simulink model "parte4_1"  (R2021b)
settings: Solver=FixedStepDiscrete  StartTime=0.0  StopTime=20  FixedStep=.03  RelTol=1e-3  EnableMultiTasking=on
PostLoadFcn:
  | try,
  | codertarget.arduinobase.registry.setBaudRate(gcs,115200)
  | disp('baud rate set to 115200 for external mode hardware serial')
  | baudrate='set_to_115200'
  | catch
  | disp('baud rate setting not needed in this version')
  | end
undefined symbols (not defined in the file): DiscIntNeverNeededParam, EncCov, h, L, Lc
libraries: MinSegLibrary_M2V5 x2, simulink x1
settings Model: SimulationMode=external  ExtModeTrigDuration=2  Creator=Alec  LastModifiedBy=Dylan
settings SolverCC: AlgebraicLoopSolver=TrustRegion
settings DataIOCC: LimitDataPoints=on  SaveFormat=Array  ReturnWorkspaceOutputs=off
settings OptimizationCC: EnhancedBackFolding=on  PassReuseOutputArgsAs=Individual arguments  ExpressionDepthLimit=2147483647  ZeroExternalMemoryAtStartup=off  ZeroInternalMemoryAtStartup=off  MaxStackSize=64  OptimizeBlockOrder=speed  DifferentSizesBufferReuse=on  OptimizationCustomize=off  EfficientTunableParamExpr=on
settings DebuggingCC: UnderspecifiedInitializationDetection=Classic  MergeDetectMultiDrivingBlocksExec=none  ParameterTunabilityLossMsg=error  StateNameClashWarn=warning  SFUnexpectedBacktrackingDiag=warning  SFNoUnconditionalDefaultTransitionDiag=warning  SFExecutionAtInitializationDiag=none  SFMachineParentedDataDiag=warning  ArithmeticOperatorsInVariantConditions=warning
settings HardwareCC: ProdBitPerInt=16  ProdBitPerPointer=16  ProdBitPerSizeT=16  ProdBitPerPtrDiffT=16  ProdLargestAtomicFloat=None  ProdWordSize=8  ProdHWDeviceType=Atmel->AVR
settings ModelReferenceCC: PropagateSignalLabelsOutOfModel=off
settings SFSimCC: SimUseLocalCustomCode=off  MATLABDynamicMemAlloc=off  CustomCodeUndefinedFunction=UseInterfaceOnly
settings RTWCC: Description=Embedded Coder  SystemTargetFile=ert.tlc  HardwareBoard=Arduino Mega 2560  TemplateMakefile=ert_default_tmf  RTWVerbose=off  RTWUseLocalCustomCode=off  Toolchain=Arduino AVR  BuildConfiguration=Faster Runs
settings CodeAppCC: ForceParamTrailComments=on  IgnoreCustomStorageClasses=off  OperatorAnnotations=on  SimulinkDataObjDesc=on  SFDataObjDesc=on  CustomSymbolStrType=$N$R$M  InsertBlockDesc=on  InternalIdentifier=Classic
settings ERTTargetCC: SupportContinuousTime=on  SupportVariableSizeSignals=on  ExtModeTransport=3  ExtModeStaticAlloc=on  ExtModeStaticAllocSize=2048  ExtModeMexFile=ext_xcp  ExtModeIntrfLevel=Level2 - Open
settings ConfigComp: CovMetricSettings=dw  CovSaveCumulativeToWorkspaceVar=on  CovSaveSingleToWorkspaceVar=on  CovExternalEMLEnable=off

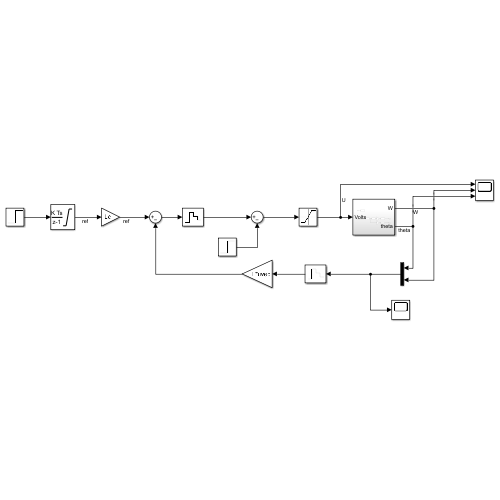
[thumbnail: Simulink's stored preview of the top-level diagram]
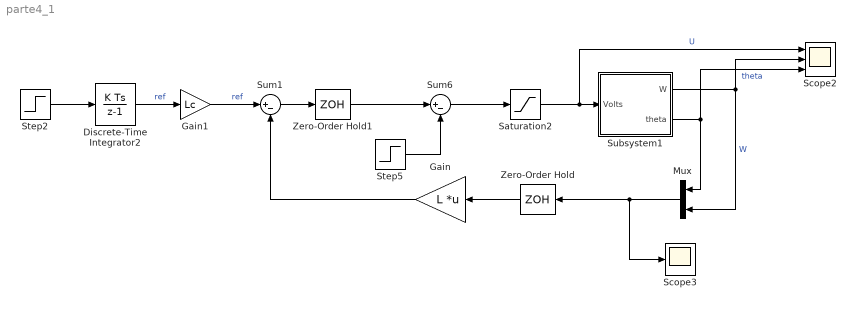
== system parte4_1 ==
  Discrete-Time Integrator2 : DiscreteIntegrator  SampleTime=h  LimitOutput=on  UpperSaturationLimit=50  LowerSaturationLimit=-50  ICPrevOutput=DiscIntNeverNeededParam  ICPrevScaledInput=DiscIntNeverNeededParam
  Gain : Gain  Gain=L  Multiplication=Matrix(K*u) (u vector)
  Gain1 : Gain  Gain=Lc
  Mux : Mux  Inputs=2
  Saturation2 : Saturate  UpperLimit=4.8  LowerLimit=-4.8
  Scope2 : Scope  NumInputPorts=3
  Scope3 : Scope
  Step2 : Step  After=60  SampleTime=0
  Step5 : Step  Time=10  After=2  SampleTime=0
  Subsystem1 : Subsystem
  Sum1 : Sum  Inputs=|+-
  Sum6 : Sum  Inputs=|+-
  Zero-Order Hold : ZeroOrderHold  SampleTime=h
  Zero-Order Hold1 : ZeroOrderHold  SampleTime=h
  wires:
  Subsystem1/2(theta) -> Mux/1, Scope2/3  "theta"
  Gain/1 -> Sum1/2
  Zero-Order Hold/1 -> Gain/1
  Step2/1 -> Discrete-Time Integrator2/1
  Saturation2/1 -> Subsystem1/1(Volts), Scope2/1  "U"
  Discrete-Time Integrator2/1 -> Gain1/1  "ref"
  Zero-Order Hold1/1 -> Sum6/1
  Subsystem1/1(W) -> Mux/2, Scope2/2  "W"
  Step5/1 -> Sum6/2
  Mux/1 -> Scope3/1, Zero-Order Hold/1
  Gain1/1 -> Sum1/1  "ref"
  Sum6/1 -> Saturation2/1
  Sum1/1 -> Zero-Order Hold1/1

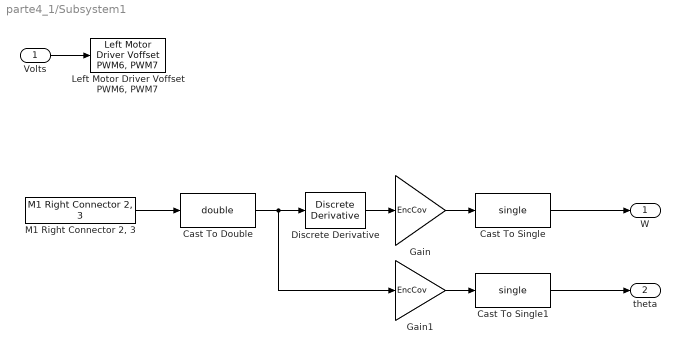
== system parte4_1/Subsystem1 ==
  Volts : Inport
  Cast To Double : DataTypeConversion  OutDataTypeStr=double
  Cast To Single : DataTypeConversion  OutDataTypeStr=single
  Cast To Single1 : DataTypeConversion  OutDataTypeStr=single
  Discrete Derivative : simulink/Discrete/Discrete Derivative  gainval=1.0  ICPrevScaledInput=0.0  OutMin=[]  OutMax=[]  OutDataType=fixdt(1, 16)  OutScaling=2^-10  DoSatur=off
  Gain : Gain  Gain=EncCov
  Gain1 : Gain  Gain=EncCov
  "Left Motor Driver Voffset PWM6, PWM7" : MinSegLibrary_M2V5/Left Motor Driver Voffset PWM6, PWM7  Vsupply=4.8  Voffset=0
      settings: SourceProductName=Rensselaer Arduino Support Package
  "M1 Right Connector 2, 3" : MinSegLibrary_M2V5/M1 Right Connector 2, 3  Encoder=0  PinA=2  PinB=3
      settings: SourceProductName=Rensselaer Arduino Support Package
  W : Outport
  theta : Outport  Port=2
  wires:
  Cast To Single/1 -> W/1
  Gain1/1 -> Cast To Single1/1
  Cast To Single1/1 -> theta/1
  "M1 Right Connector 2, 3"/1 -> Cast To Double/1
  Cast To Double/1 -> Gain1/1, Discrete Derivative/1
  Volts/1 -> "Left Motor Driver Voffset PWM6, PWM7"/1
  Discrete Derivative/1 -> Gain/1
  Gain/1 -> Cast To Single/1
